simulink subsystem "ApplFOCSLHighPrio"  (R2024b)
settings: Solver=VariableStepAuto  StartTime=0.0  StopTime=10.0  RelTol=1e-3
values from neighbouring files (symbols this model uses):
  Ts = 2 * T_pwm    (= 0.0001)    [s32k344Data.m]
undefined symbols (not defined in the file or in its folder): inverter, pmsm, PU_System
libraries: mcbcontrolslib x5, mcbpositiondecoderlib x3, mcbsensorlessestimatorlib x2, mcbfoclib x1, mcbpmsmiflib x1
settings Model: Creator=The MathWorks, Inc.  LastModifiedBy=nxf64875
settings RTWCC: GPUComputeCapability=3.5  LargeConstantGeneration=WriteOnlyDNNConstantsToDataFiles

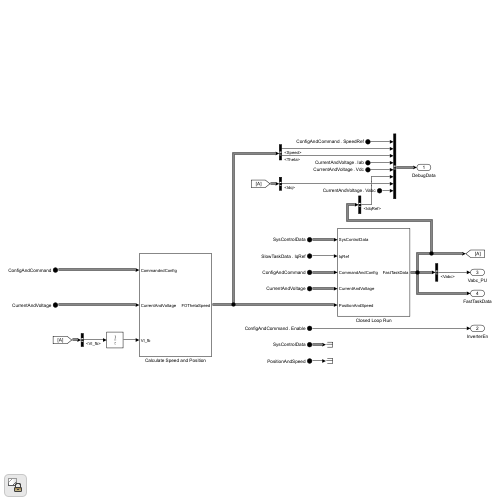
[thumbnail: Simulink's stored preview of the top-level diagram]
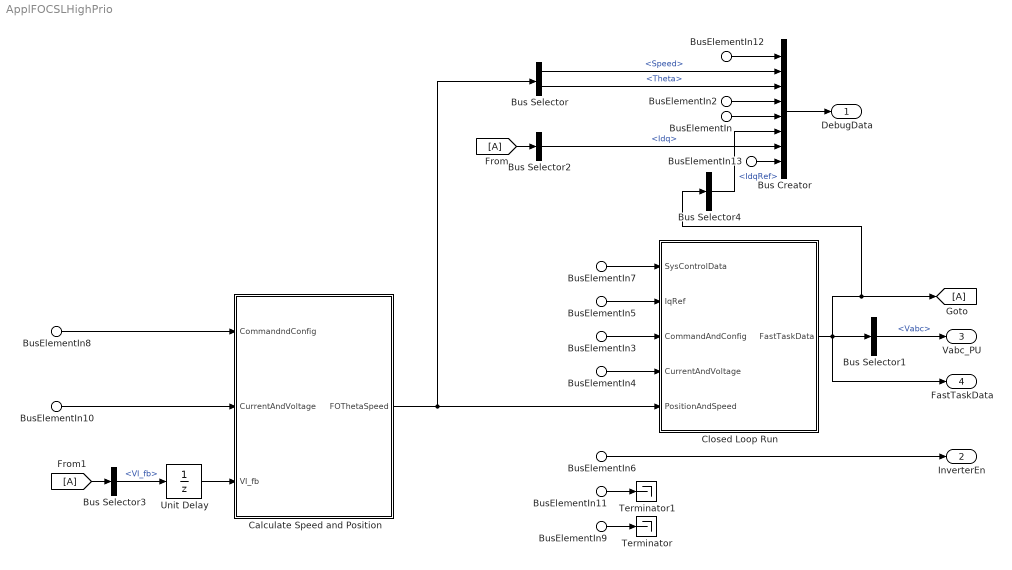
== system ApplFOCSLHighPrio ==
  BusElementIn3 : Inport  PortName=ConfigAndCommand
  BusElementIn8 : Inport  PortName=ConfigAndCommand
  BusElementIn6 : Inport  PortName=ConfigAndCommand  Element=Enable
  BusElementIn12 : Inport  PortName=ConfigAndCommand  Element=SpeedRef
  BusElementIn4 : Inport  Port=2  PortName=CurrentAndVoltage
  BusElementIn10 : Inport  Port=2  PortName=CurrentAndVoltage
  BusElementIn2 : Inport  Port=2  PortName=CurrentAndVoltage  Element=Iab
  BusElementIn : Inport  Port=2  PortName=CurrentAndVoltage  Element=Vdc
  BusElementIn13 : Inport  Port=2  PortName=CurrentAndVoltage  Element=Vabc
  BusElementIn9 : Inport  Port=3  PortName=PositionAndSpeed
  BusElementIn5 : Inport  Port=4  PortName=SlowTaskData  Element=IqRef
  BusElementIn7 : Inport  Port=5  PortName=SysControlData
  BusElementIn11 : Inport  Port=5  PortName=SysControlData
  Bus Creator : BusCreator  Inputs=8
  Bus Selector : BusSelector  OutputSignals=Speed,Theta
  Bus Selector1 : BusSelector  OutputSignals=Vabc
  Bus Selector2 : BusSelector  OutputSignals=Idq
  Bus Selector3 : BusSelector  OutputSignals=VI_fb
  Bus Selector4 : BusSelector  OutputSignals=IdqRef
  Calculate Speed and Position : Subsystem
  Closed Loop Run : Subsystem
  From : From
  From1 : From
  Goto : Goto
  Terminator : Terminator
  Terminator1 : Terminator
  Unit Delay : UnitDelay  SampleTime=-1  HasFrameUpgradeWarning=on
  DebugData : Outport
  InverterEn : Outport  Port=2
  Vabc_PU : Outport  Port=3
  FastTaskData : Outport  Port=4
  wires:
  Bus Selector3/1 -> Unit Delay/1  "<VI_fb>"
  From1/1 -> Bus Selector3/1
  From/1 -> Bus Selector2/1
  BusElementIn13/1 -> Bus Creator/8
  Bus Selector2/1 -> Bus Creator/7  "<Idq>"
  BusElementIn/1 -> Bus Creator/5
  Bus Selector/2 -> Bus Creator/3  "<Theta>"
  Bus Selector/1 -> Bus Creator/2  "<Speed>"
  BusElementIn12/1 -> Bus Creator/1
  BusElementIn11/1 -> Terminator1/1
  Unit Delay/1 -> Calculate Speed and Position/3(VI_fb)
  BusElementIn10/1 -> Calculate Speed and Position/2(CurrentAndVoltage)
  BusElementIn8/1 -> Calculate Speed and Position/1(CommandndConfig)
  Calculate Speed and Position/1(FOThetaSpeed) -> Bus Selector/1, Closed Loop Run/5(PositionAndSpeed)
  BusElementIn9/1 -> Terminator/1
  BusElementIn7/1 -> Closed Loop Run/1(SysControlData)
  BusElementIn6/1 -> InverterEn/1
  Bus Selector1/1 -> Vabc_PU/1  "<Vabc>"
  BusElementIn4/1 -> Closed Loop Run/4(CurrentAndVoltage)
  BusElementIn5/1 -> Closed Loop Run/2(IqRef)
  BusElementIn3/1 -> Closed Loop Run/3(CommandAndConfig)
  Closed Loop Run/1(FastTaskData) -> FastTaskData/1, Goto/1, Bus Selector4/1, Bus Selector1/1
  Bus Creator/1 -> DebugData/1
  BusElementIn2/1 -> Bus Creator/4
  Bus Selector4/1 -> Bus Creator/6  "<IdqRef>"

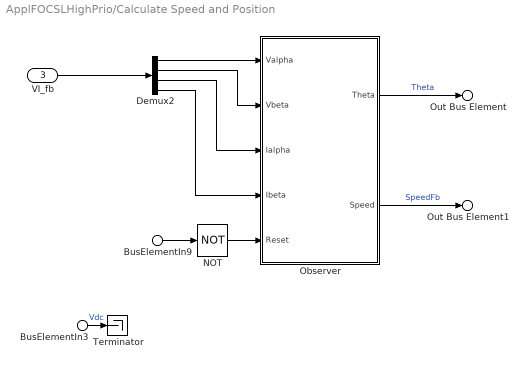
== system ApplFOCSLHighPrio/Calculate Speed and Position ==
  BusElementIn9 : Inport  PortName=CommandndConfig  Element=Enable
  BusElementIn3 : Inport  Port=2  PortName=CurrentAndVoltage  Element=Vdc
  VI_fb : Inport  Port=3
  Demux2 : Demux
  NOT : Logic  Operator=NOT  IconShape=distinctive  AllPortsSameDT=off  OutDataTypeStr=boolean
  Observer : Subsystem  Variant=on
  Terminator : Terminator
  Out Bus Element : Outport  PortName=FOThetaSpeed  Element=Theta
  Out Bus Element1 : Outport  PortName=FOThetaSpeed  Element=Speed
  wires:
  VI_fb/1 -> Demux2/1
  BusElementIn3/1 -> Terminator/1  "Vdc"
  Demux2/4 -> Observer/4(Ibeta)
  Demux2/3 -> Observer/3(Ialpha)
  Demux2/2 -> Observer/2(Vbeta)
  Demux2/1 -> Observer/1(Valpha)
  Observer/2(Speed) -> Out Bus Element1/1  "SpeedFb"
  Observer/1(Theta) -> Out Bus Element/1  "Theta"
  NOT/1 -> Observer/5(Reset)
  BusElementIn9/1 -> NOT/1

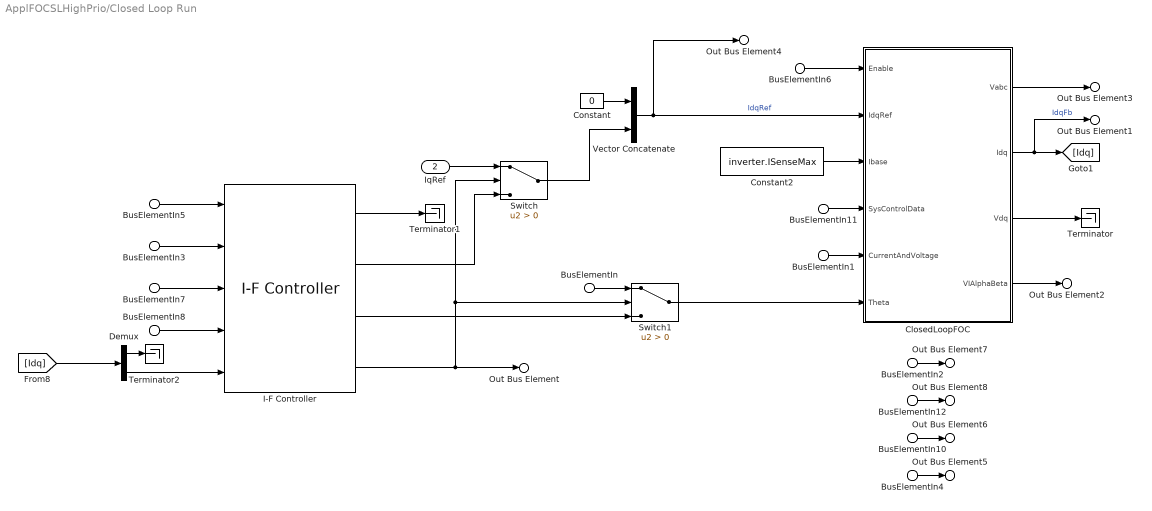
== system ApplFOCSLHighPrio/Closed Loop Run ==
  BusElementIn11 : Inport  PortName=SysControlData
  BusElementIn7 : Inport  PortName=SysControlData  Element=SpeedRef
  IqRef : Inport  Port=2
  BusElementIn2 : Inport  Port=3  PortName=CommandAndConfig  Element=SpeedRef
  BusElementIn12 : Inport  Port=3  PortName=CommandAndConfig  Element=Enable
  BusElementIn5 : Inport  Port=3  PortName=CommandAndConfig  Element=Enable
  BusElementIn6 : Inport  Port=3  PortName=CommandAndConfig  Element=Enable
  BusElementIn1 : Inport  Port=4  PortName=CurrentAndVoltage
  BusElementIn4 : Inport  Port=5  PortName=PositionAndSpeed  Element=Speed
  BusElementIn8 : Inport  Port=5  PortName=PositionAndSpeed  Element=Speed
  BusElementIn10 : Inport  Port=5  PortName=PositionAndSpeed  Element=Theta
  BusElementIn : Inport  Port=5  PortName=PositionAndSpeed  Element=Theta
  BusElementIn3 : Inport  Port=5  PortName=PositionAndSpeed  Element=Theta
  ClosedLoopFOC : Subsystem
  Constant : Constant  Value=0  OutDataTypeStr=single
  Constant2 : Constant  Value=inverter.ISenseMax  OutDataTypeStr=dataType
  Demux : Demux  Outputs=2
  I-F Controller : mcbpmsmiflib/I-F Controller  EnableSpeedDamp=off  PolePairs=pmsm.p  PositionUnit=Per-unit  SpeedUnit=Per-unit  PerUnitSpeed=PU_System.N_base  CurrentUnit=Per-unit  TempCurrentUnit=Per-unit  MaxStatorCurrent=PU_System.I_base  BlkSampleTime=Ts  ParameterBusInput=off  OlClSpeed=pmsm.OL2CL  ClOlSpeed=pmsm.CL2OL  MaxStartingCurrent=pmsm.I_rated * 0.5  MaxAcceleration=PU_System.N_base / 10  CurrentDownSlope=pmsm.I_rated * 10  IdleTime=1  Angle=0.1745  VoltageUnit=SI unit  TempVoltageUnit=SI unit  MaxStatorVoltage=13.8564  DampCoeff=2.6172
  Switch : Switch  Criteria=u2 > Threshold  SaturateOnIntegerOverflow=off  InputSameDT=off
  Switch1 : Switch  Criteria=u2 > Threshold  SaturateOnIntegerOverflow=off  InputSameDT=off
  Terminator : Terminator
  Terminator1 : Terminator
  Terminator2 : Terminator
  Vector Concatenate : Concatenate
  Out Bus Element : Outport  PortName=FastTaskData  Element=EnClosedLoop
  Out Bus Element1 : Outport  PortName=FastTaskData  Element=Idq
  Out Bus Element2 : Outport  PortName=FastTaskData  Element=VI_fb
  Out Bus Element3 : Outport  PortName=FastTaskData  Element=Vabc
  Out Bus Element4 : Outport  PortName=FastTaskData  Element=IdqRef
  Out Bus Element5 : Outport  PortName=FastTaskData  Element=Speed
  Out Bus Element6 : Outport  PortName=FastTaskData  Element=Theta
  Out Bus Element7 : Outport  PortName=FastTaskData  Element=SpeedRef
  Out Bus Element8 : Outport  PortName=FastTaskData  Element=Enable
  wires:
  I-F Controller/2 -> Switch/3
  BusElementIn7/1 -> I-F Controller/3
  Demux/2 -> I-F Controller/5
  I-F Controller/3 -> Switch1/3
  BusElementIn8/1 -> I-F Controller/4
  I-F Controller/4 -> Out Bus Element/1, Switch1/2, Switch/2
  BusElementIn5/1 -> I-F Controller/1
  BusElementIn3/1 -> I-F Controller/2
  Demux/1 -> Terminator2/1
  Switch1/1 -> ClosedLoopFOC/6(Theta)
  Switch/1 -> Vector Concatenate/2
  BusElementIn/1 -> Switch1/1
  IqRef/1 -> Switch/1
  Constant/1 -> Vector Concatenate/1
  I-F Controller/1 -> Terminator1/1
  ClosedLoopFOC/1(Vabc) -> Out Bus Element3/1
  BusElementIn6/1 -> ClosedLoopFOC/1(Enable)
  ClosedLoopFOC/2(Idq) -> Out Bus Element1/1, [Idq]  "IdqFb"
  ClosedLoopFOC/4(VIAlphaBeta) -> Out Bus Element2/1
  BusElementIn11/1 -> ClosedLoopFOC/4(SysControlData)
  Vector Concatenate/1 -> ClosedLoopFOC/2(IdqRef), Out Bus Element4/1  "IdqRef"
  ClosedLoopFOC/3(Vdq) -> Terminator/1
  Constant2/1 -> ClosedLoopFOC/3(Ibase)
  BusElementIn4/1 -> Out Bus Element5/1
  BusElementIn1/1 -> ClosedLoopFOC/5(CurrentAndVoltage)
  [Idq] -> Demux/1
  BusElementIn10/1 -> Out Bus Element6/1
  BusElementIn2/1 -> Out Bus Element7/1
  BusElementIn12/1 -> Out Bus Element8/1

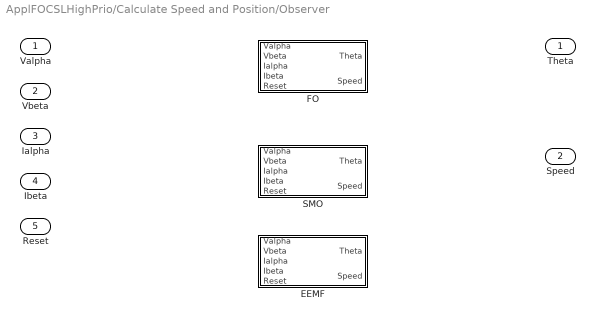
== system ApplFOCSLHighPrio/Calculate Speed and Position/Observer ==
  Valpha : Inport
  Vbeta : Inport  Port=2
  Ialpha : Inport  Port=3
  Ibeta : Inport  Port=4
  Reset : Inport  Port=5
  EEMF : Subsystem  VariantControl=strcmp(pmsm.Sensor, 'EEMF')
  FO : Subsystem  VariantControl=strcmp(pmsm.Sensor, 'FO')
  SMO : Subsystem  VariantControl=strcmp(pmsm.Sensor, 'SMO')
  Theta : Outport
  Speed : Outport  Port=2

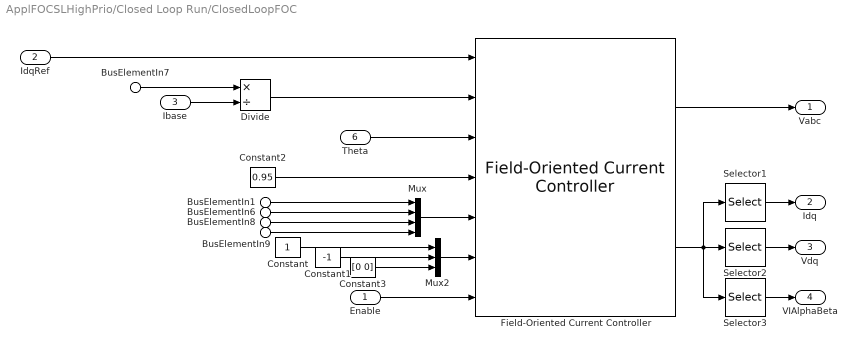
== system ApplFOCSLHighPrio/Closed Loop Run/ClosedLoopFOC ==
  Enable : Inport
  IdqRef : Inport  Port=2
  Ibase : Inport  Port=3
  BusElementIn1 : Inport  Port=4  PortName=SysControlData  Element=PIGains.Daxis_Kp
  BusElementIn6 : Inport  Port=4  PortName=SysControlData  Element=PIGains.Daxis_Ki*Ts
  BusElementIn8 : Inport  Port=4  PortName=SysControlData  Element=PIGains.Qaxis_Kp
  BusElementIn9 : Inport  Port=4  PortName=SysControlData  Element=PIGains.Qaxis_Ki*Ts
  BusElementIn7 : Inport  Port=5  PortName=CurrentAndVoltage  Element=Iab
  Theta : Inport  Port=6
  Constant : Constant  OutDataTypeStr=single
  Constant1 : Constant  Value=-1  OutDataTypeStr=single
  Constant2 : Constant  Value=0.95  OutDataTypeStr=single
  Constant3 : Constant  Value=[0 0]  OutDataTypeStr=single
  Divide : Product  Inputs=*/
  Field-Oriented Current Controller : mcbfoclib/Field-Oriented Current Controller  AngleUnit=Per-unit  NumberOfLUTPoints=1024  AxisAlignment=D-axis  SaturationMethod=D-Q equivalence  PWMMethod=SVM: space vector modulation
  Mux : Mux
  Mux2 : Mux  Inputs=3
  Selector1 : Selector  InputPortWidth=8  IndexOptions=Index vector (dialog)  Indices=[1 2]  OutputSizes=1
  Selector2 : Selector  InputPortWidth=8  IndexOptions=Index vector (dialog)  Indices=[3 4]  OutputSizes=1
  Selector3 : Selector  InputPortWidth=8  IndexOptions=Index vector (dialog)  Indices=[5 6 7 8]  OutputSizes=1
  Vabc : Outport
  Idq : Outport  Port=2
  Vdq : Outport  Port=3
  VIAlphaBeta : Outport  Port=4
  wires:
  Mux/1 -> Field-Oriented Current Controller/5
  Theta/1 -> Field-Oriented Current Controller/3
  Enable/1 -> Field-Oriented Current Controller/7
  Constant2/1 -> Field-Oriented Current Controller/4
  Selector3/1 -> VIAlphaBeta/1
  Selector2/1 -> Vdq/1
  Constant1/1 -> Mux2/2
  IdqRef/1 -> Field-Oriented Current Controller/1
  Selector1/1 -> Idq/1
  Field-Oriented Current Controller/1 -> Vabc/1
  Ibase/1 -> Divide/2
  Divide/1 -> Field-Oriented Current Controller/2
  BusElementIn7/1 -> Divide/1
  Constant/1 -> Mux2/1
  Constant3/1 -> Mux2/3
  Mux2/1 -> Field-Oriented Current Controller/6
  Field-Oriented Current Controller/2 -> Selector1/1, Selector3/1, Selector2/1
  BusElementIn1/1 -> Mux/1
  BusElementIn6/1 -> Mux/2
  BusElementIn8/1 -> Mux/3
  BusElementIn9/1 -> Mux/4

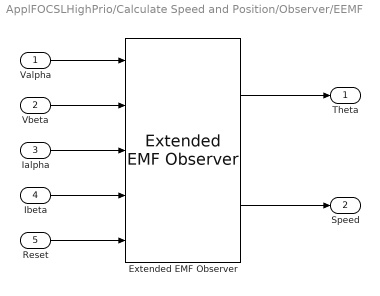
== system ApplFOCSLHighPrio/Calculate Speed and Position/Observer/EEMF ==
  Valpha : Inport
  Vbeta : Inport  Port=2
  Ialpha : Inport  Port=3
  Ibeta : Inport  Port=4
  Reset : Inport  Port=5
  Extended EMF Observer : mcbsensorlessestimatorlib/Extended EMF Observer  InputUnit=Per-unit  PosOut=Electrical position  BlkSampleTime=Ts  StatorResistance=pmsm.Rs + inverter.R_board  StatorDaxisInductance=pmsm.Ld  StatorQaxisInductance=pmsm.Lq  MaxApplicationSpeed=pmsm.N_rated * 2  PolePairs=pmsm.p  MaxStatorVoltage=inverter.V_dc/sqrt(3)  MaxStatorCurrent=inverter.ISenseMax  Alpha=10  EEMFCutoffFreq="pmsm.N_base  / 60 * pmsm.p * 10"  Kp=250  Ki=200000  N_points=1024  SpeedCutoffFreq=pmsm.N_base / 60 * pmsm.p * 0.2  PositionUnit=Per-unit  PositionDataType=dataType  SpeedUnit=RPM  PerUnitSpeed=PU_System.N_base  SpeedDataType=dataType  TableDatatype=dataType
  Theta : Outport
  Speed : Outport  Port=2
  wires:
  Extended EMF Observer/2 -> Speed/1
  Valpha/1 -> Extended EMF Observer/1
  Extended EMF Observer/1 -> Theta/1
  Vbeta/1 -> Extended EMF Observer/2
  Ialpha/1 -> Extended EMF Observer/3
  Ibeta/1 -> Extended EMF Observer/4
  Reset/1 -> Extended EMF Observer/5

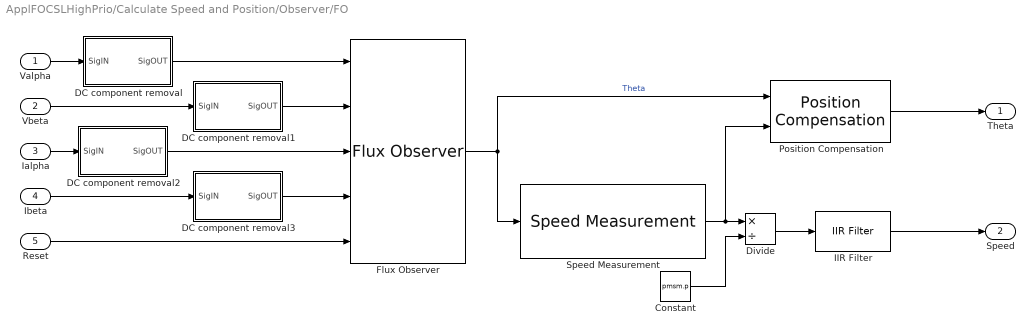
== system ApplFOCSLHighPrio/Calculate Speed and Position/Observer/FO ==
  Valpha : Inport
  Vbeta : Inport  Port=2
  Ialpha : Inport  Port=3
  Ibeta : Inport  Port=4
  Reset : Inport  Port=5
  Constant : Constant  Value=pmsm.p  OutDataTypeStr=Inherit: Inherit via back propagation
  DC component removal : Subsystem
  DC component removal1 : Subsystem
  DC component removal2 : Subsystem
  DC component removal3 : Subsystem
  Divide : Product  Inputs=*/  RndMeth=Simplest  OutDataTypeStr=Inherit: Same as first input
  Flux Observer : mcbpositiondecoderlib/Flux Observer  MotorSelection=PMSM  DataTypeSelect=off  BlockInputUnit=Per-unit  PerUnitVoltage=12/sqrt(3)  PerUnitCurrent=inverter.ISenseMax  PositionSelect=on  FluxSelect=off  TorqueSelect=off  PolePairs=4  StatorResistance=pmsm.Rs  StatorDAxisInductance=pmsm.Ld  StatorLeakageInductance=0.0068  RotorLeakageInductance=0.0068  MagnetizingInductance=0.0300  CutoffFreq=pmsm.N_base * pmsm.p / 60 * 0.09  BlockSampleTime=Ts  ParameterBusInput=off  PositionUnit=Per-unit  PositionDatatype=single  FluxUnit=Weber  PerUnitFlux=0.1  FluxDatatype=single  TorqueUnit=Nm  PerUnitTorque=100  TorqueDatatype=single  DataType=0
  IIR Filter : mcbcontrolslib/IIR Filter  VariantControl=Low Pass Filter  VariantSelect=Low-pass  FilterConstantInputType=Specify via dialog  Filter_constant=0.01  advancedSettings=off  Ts=50e-6  cutOff_freq=32.1525
  Position Compensation : mcbpositiondecoderlib/Position Compensation  PhaseCompensationType=High-pass filter delay  OffsetValue=0.1  CutOffFreq=16  NumberSampleDelay=1  BlkSampleTime=50e-6  PositionUnit=Per unit  SpeedUnit=RPM  MaximumApplicationSpeed=10000
  Speed Measurement : mcbpositiondecoderlib/Speed Measurement  PositionUnit=Per unit  PositionScalingDatatype=uint32  SpeedCalculationMode=Time interval for speed calculation  SampleTimeAsync=Ts  MaximumApplicationSpeed=6000  SpeedResolution=5e-6  DelayLength=10  MaximumMeasurableSpeed=29999  MeasurableSpeedResolution=1.397e-05  SpeedUnit=RPM  PerUnitSpeed=4000  SpeedDataType=dataType
  Theta : Outport
  Speed : Outport  Port=2
  wires:
  Ibeta/1 -> DC component removal3/1(SigIN)
  IIR Filter/1 -> Speed/1
  Vbeta/1 -> DC component removal1/1(SigIN)
  Ialpha/1 -> DC component removal2/1(SigIN)
  Position Compensation/1 -> Theta/1
  Valpha/1 -> DC component removal/1(SigIN)
  Reset/1 -> Flux Observer/5
  Divide/1 -> IIR Filter/1
  Speed Measurement/1 -> Position Compensation/2, Divide/1
  Constant/1 -> Divide/2
  Flux Observer/1 -> Speed Measurement/1, Position Compensation/1  "Theta"
  DC component removal/1(SigOUT) -> Flux Observer/1
  DC component removal1/1(SigOUT) -> Flux Observer/2
  DC component removal2/1(SigOUT) -> Flux Observer/3
  DC component removal3/1(SigOUT) -> Flux Observer/4

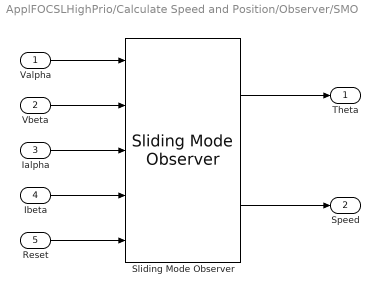
== system ApplFOCSLHighPrio/Calculate Speed and Position/Observer/SMO ==
  Valpha : Inport
  Vbeta : Inport  Port=2
  Ialpha : Inport  Port=3
  Ibeta : Inport  Port=4
  Reset : Inport  Port=5
  Sliding Mode Observer : mcbsensorlessestimatorlib/Sliding Mode Observer  InputUnit=Per-unit  BlkSampleTime=Ts  StatorResistance=pmsm.Rs  StatorInductance=pmsm.Ld  MaxApplicationSpeed=pmsm.N_base  PolePairs=pmsm.p  MaxStatorVoltage=inverter.V_dc/sqrt(3)  MaxStatorCurrent=inverter.ISenseMax  DisturbanceObserverGain=0.9  CurrentObserverGain=0.14634  CutoffFreq=1006.8  PositionUnit=Per unit  PositionDataType=dataType  SpeedUnit=RPM  PerUnitSpeed=1000  SpeedDataType=dataType
  Theta : Outport
  Speed : Outport  Port=2
  wires:
  Ibeta/1 -> Sliding Mode Observer/4
  Sliding Mode Observer/2 -> Speed/1
  Vbeta/1 -> Sliding Mode Observer/2
  Ialpha/1 -> Sliding Mode Observer/3
  Sliding Mode Observer/1 -> Theta/1
  Valpha/1 -> Sliding Mode Observer/1
  Reset/1 -> Sliding Mode Observer/5

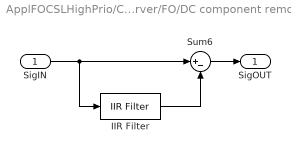
== system ApplFOCSLHighPrio/Calculate Speed and Position/Observer/FO/DC component removal ==
  SigIN : Inport
  IIR Filter : mcbcontrolslib/IIR Filter  VariantControl=Low Pass Filter  VariantSelect=Low-pass  FilterConstantInputType=Specify via dialog  Filter_constant=0.005*(Ts/50e-6)  advancedSettings=off  Ts=50e-6  cutOff_freq=32.1525
  Sum6 : Sum  Inputs=|+-  RndMeth=Simplest  OutDataTypeStr=Inherit: Same as first input
  SigOUT : Outport
  wires:
  IIR Filter/1 -> Sum6/2
  SigIN/1 -> IIR Filter/1, Sum6/1
  Sum6/1 -> SigOUT/1

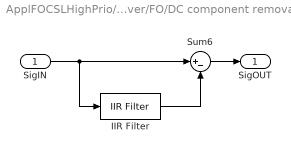
== system ApplFOCSLHighPrio/Calculate Speed and Position/Observer/FO/DC component removal1 ==
  SigIN : Inport
  IIR Filter : mcbcontrolslib/IIR Filter  VariantControl=Low Pass Filter  VariantSelect=Low-pass  FilterConstantInputType=Specify via dialog  Filter_constant=0.005*(Ts/50e-6)  advancedSettings=off  Ts=50e-6  cutOff_freq=32.1525
  Sum6 : Sum  Inputs=|+-  RndMeth=Simplest  OutDataTypeStr=Inherit: Same as first input
  SigOUT : Outport
  wires:
  Sum6/1 -> SigOUT/1
  SigIN/1 -> Sum6/1, IIR Filter/1
  IIR Filter/1 -> Sum6/2

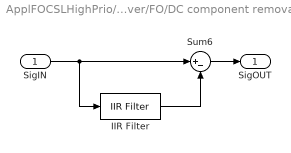
== system ApplFOCSLHighPrio/Calculate Speed and Position/Observer/FO/DC component removal2 ==
  SigIN : Inport
  IIR Filter : mcbcontrolslib/IIR Filter  VariantControl=Low Pass Filter  VariantSelect=Low-pass  FilterConstantInputType=Specify via dialog  Filter_constant=0.005*(Ts/50e-6)  advancedSettings=off  Ts=50e-6  cutOff_freq=32.1525
  Sum6 : Sum  Inputs=|+-  RndMeth=Simplest  OutDataTypeStr=Inherit: Same as first input
  SigOUT : Outport
  wires:
  IIR Filter/1 -> Sum6/2
  SigIN/1 -> IIR Filter/1, Sum6/1
  Sum6/1 -> SigOUT/1

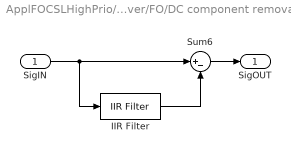
== system ApplFOCSLHighPrio/Calculate Speed and Position/Observer/FO/DC component removal3 ==
  SigIN : Inport
  IIR Filter : mcbcontrolslib/IIR Filter  VariantControl=Low Pass Filter  VariantSelect=Low-pass  FilterConstantInputType=Specify via dialog  Filter_constant=0.005*(Ts/50e-6)  advancedSettings=off  Ts=50e-6  cutOff_freq=32.1525
  Sum6 : Sum  Inputs=|+-  RndMeth=Simplest  OutDataTypeStr=Inherit: Same as first input
  SigOUT : Outport
  wires:
  Sum6/1 -> SigOUT/1
  SigIN/1 -> Sum6/1, IIR Filter/1
  IIR Filter/1 -> Sum6/2
